simulink subsystem "rollOuterLoop"  (R2026a)
settings: Solver=VariableStepAuto
values from neighbouring files (symbols this model uses):
  outerLoopParams = 0.5    [controllerParams.sldd]
settings Model: DataDictionary=controllerParams.sldd  EnableAccessToBaseWorkspace=off  Creator=maxhu  LastModifiedBy=maxhu

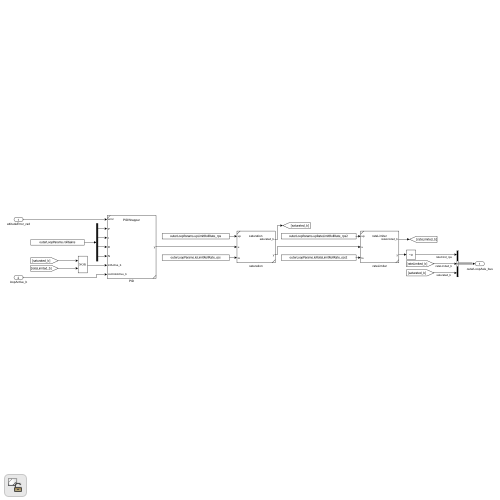
[thumbnail: Simulink's stored preview of the top-level diagram]
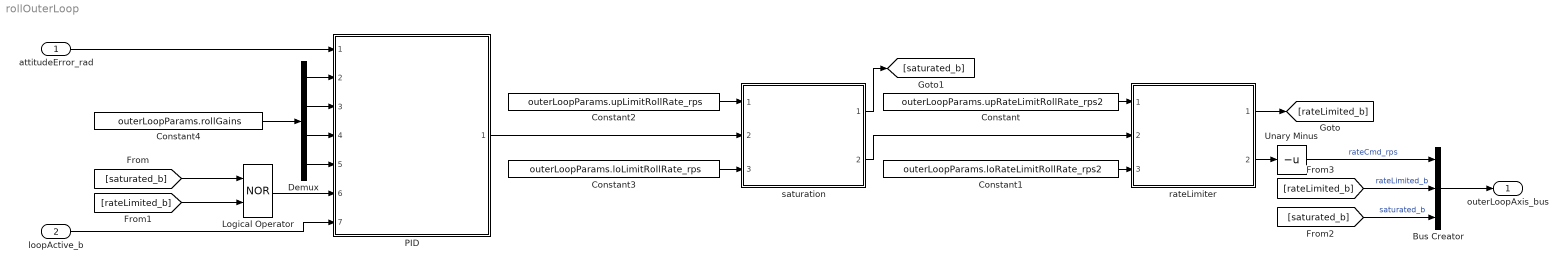
== system rollOuterLoop ==
  attitudeError_rad : Inport
  loopActive_b : Inport  Port=2
  Bus Creator : BusCreator  Inputs=3
  Constant : Constant  Value=outerLoopParams.upRateLimitRollRate_rps2
  Constant1 : Constant  Value=outerLoopParams.loRateLimitRollRate_rps2
  Constant2 : Constant  Value=outerLoopParams.upLimitRollRate_rps
  Constant3 : Constant  Value=outerLoopParams.loLimitRollRate_rps
  Constant4 : Constant  Value=outerLoopParams.rollGains
  Demux : Demux
  Logical Operator : Logic  Operator=NOR  AllPortsSameDT=off  OutDataTypeStr=boolean
  PID : Subsystem  ReferencedSubsystem=PIDWrapper
  Unary Minus : UnaryMinus
  rateLimiter : Subsystem  ReferencedSubsystem=rateLimiter
  saturation : Subsystem  ReferencedSubsystem=saturation
  outerLoopAxis_bus : Outport
  wires:
  Logical Operator/1 -> PID/6
  attitudeError_rad/1 -> PID/1
  [rateLimited_b] -> Logical Operator/2
  [saturated_b] -> Logical Operator/1
  Demux/1 -> PID/2
  Demux/4 -> PID/5
  Demux/3 -> PID/4
  Demux/2 -> PID/3
  Constant4/1 -> Demux/1
  [saturated_b] -> Bus Creator/3  "saturated_b"
  Bus Creator/1 -> outerLoopAxis_bus/1
  [rateLimited_b] -> Bus Creator/2  "rateLimited_b"
  Constant2/1 -> saturation/1
  Constant3/1 -> saturation/3
  PID/1 -> saturation/2
  saturation/1 -> [saturated_b]
  Constant/1 -> rateLimiter/1
  Constant1/1 -> rateLimiter/3
  rateLimiter/1 -> [rateLimited_b]
  saturation/2 -> rateLimiter/2
  loopActive_b/1 -> PID/7
  rateLimiter/2 -> Unary Minus/1
  Unary Minus/1 -> Bus Creator/1  "rateCmd_rps"
